simulink model "TormoziRastgard"  (R2014a)
settings: Solver=ode45  StartTime=0.0  StopTime=2  RelTol=1e-3
libraries: powerlib x13, powerlib_meascontrol x1
settings Model: Creator=pc6229  LastModifiedBy=pc6229

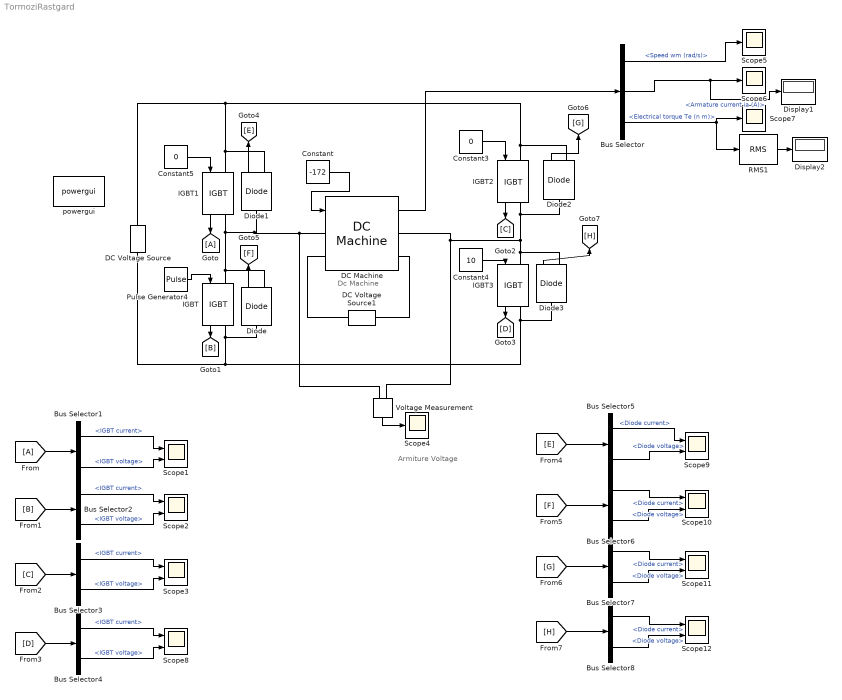
== system TormoziRastgard ==
  note: Armiture Voltage
  note: Dc Machine
  Bus Selector : BusSelector  OutputSignals=Speed wm (rad/s),Armature current ia (A),Electrical torque Te (n m)
  Bus Selector{1..4} (4 alike) : BusSelector  OutputSignals=IGBT current,IGBT voltage
  Bus Selector{5..8} (4 alike) : BusSelector  OutputSignals=Diode current,Diode voltage
  Constant : Constant  Value=-172
  Constant3 : Constant  Value=0
  Constant4 : Constant  Value=10
  Constant5 : Constant  Value=0
  DC Machine : powerlib/Machines/DC Machine  PresetModel=No  MechanicalLoad=Torque TL  FieldType=Wound  ShowDetailedParameters=on  MeasurementBus=off  RLa="[ 0.4  0.04]"  RLf=[ 95 150]  Laf=1.85  MachineConstant=Torque constant (N.m/A)  Ke=1.8  Kt=1.8  J=1  Bm=0  Tf=0  w0=1  Ifinit=1  TsPowergui=0  TsBlock=-1
  DC Voltage Source : powerlib/Electrical Sources/DC Voltage Source  Amplitude=600  Measurements=None
  DC Voltage Source1 : powerlib/Electrical Sources/DC Voltage Source  Amplitude=135  Measurements=None
  Diode{,1..3} (4 alike) : powerlib/Power Electronics/Diode  Ron=0.001  Lon=0  Vf=0.8  IC=0  UseSnubber=off  Rs=500  Cs=250e-9  Measurements=on
  Display1 : Display
  Display2 : Display
  IGBT{,1..3} (4 alike) : powerlib/Power Electronics/IGBT  Ron=0.001  Lon=0  Vf=1  Tf=1e-6  Tt=2e-6  IC=0  Rs=1e5  Cs=inf  Measurements=on
  Pulse Generator4 : DiscretePulseGenerator  PulseType=Time based  Amplitude=10  Period=0.002  PulseWidth=60
  RMS1 : powerlib_meascontrol/Measurements/RMS  TrueRMS=on  Freq=60  RMSInit=120  Ts=0
  Scope{1..3,8..12} (8 alike) : Scope  NumInputPorts=2
      Scope1 settings: YMin=-5~-5  YMax=5~5
      Scope10 settings: YMin=-5~-5  YMax=5~5  SaveName=ScopeData9
      Scope11 settings: YMin=-5~-5  YMax=5~5  SaveName=ScopeData10
      Scope12 settings: YMin=-5~-5  YMax=5~5  SaveName=ScopeData11
      Scope2 settings: YMin=-5~-5  YMax=5~5
      Scope3 settings: YMin=-5~-5  YMax=5~5  SaveName=ScopeData2
      Scope8 settings: YMin=-5~-5  YMax=5~5  SaveName=ScopeData7
      Scope9 settings: YMin=-5~-5  YMax=5~5  SaveName=ScopeData8
  Scope{4..7} (4 alike) : Scope
      Scope4 settings: SaveName=ScopeData3
      Scope5 settings: YMin=100  YMax=107.5  SaveName=ScopeData4
      Scope6 settings: TimeRange=0.01148000060583776  YMin=-90  YMax=10  SaveName=ScopeData5
      Scope7 settings: SaveName=ScopeData6
  Voltage Measurement : powerlib/Measurements/Voltage Measurement  PhasorSimulation=off  OutputType=Complex  PSBequivalent=0
  powergui : powerlib/powergui  Priority=1  SimulationMode=Discrete  SolverType=Tustin  SampleTime=50e-6  frequency=60  SPID=off  DisableSnubberDevices=off  DisableRonSwitches=off  DisableVfSwitches=off  SwTol=0  Interpol=off  DisplayEquations=off  Ts=0  methode=off  frequencyindice=0  Pbase=100e6  ErrMax=1e-4  Iterations=50  UnitsV=kV  UnitsW=MW  FunctionMessages=off  echomessages=off  HookPort=off  EnableUseOfTLC=off  x0status=blocks  RestoreLinks=warning  ResistiveCurrentMeasurement=off  Frange=[0:2:500]  Ylog=off  Xlog=on  ShowGrid=off  save=off  variable=ZData  structure=0  ZoomFFT=off  StartTime=0.0  cycles=1  DisplayStyle=1  fundamental=60  FreqAxis=off  MaxFrequency=1000  frequencyindicesteady=1  RmsSteady=1  display=off
  wires:
  Constant/1 -> DC Machine/1
  DC Machine/1 -> Bus Selector/1
  Bus Selector/1 -> Scope5/1  "<Speed wm (rad/s)>"
  Bus Selector/2 -> Display1/1, Scope6/1  "<Armature current ia (A)>"
  Constant3/1 -> IGBT2/1
  Constant4/1 -> IGBT3/1
  Bus Selector/3 -> RMS1/1, Scope7/1  "<Electrical torque Te (n m)>"
  Pulse Generator4/1 -> IGBT/1
  Constant5/1 -> IGBT1/1
  RMS1/1 -> Display2/1
  Voltage Measurement/1 -> Scope4/1
  IGBT1/1 -> [A]
  IGBT/1 -> [B]
  IGBT2/1 -> [C]
  IGBT3/1 -> [D]
  [A] -> Bus Selector1/1
  [B] -> Bus Selector2/1
  [C] -> Bus Selector3/1
  [D] -> Bus Selector4/1
  Bus Selector1/1 -> Scope1/1  "<IGBT current>"
  Bus Selector1/2 -> Scope1/2  "<IGBT voltage>"
  Bus Selector2/1 -> Scope2/1  "<IGBT current>"
  Bus Selector2/2 -> Scope2/2  "<IGBT voltage>"
  Bus Selector3/2 -> Scope3/2  "<IGBT voltage>"
  Bus Selector3/1 -> Scope3/1  "<IGBT current>"
  Bus Selector4/1 -> Scope8/1  "<IGBT current>"
  Bus Selector4/2 -> Scope8/2  "<IGBT voltage>"
  Diode1/1 -> [E]
  Diode/1 -> [F]
  Diode3/1 -> [H]
  Diode2/1 -> [G]
  [E] -> Bus Selector5/1
  [F] -> Bus Selector6/1
  [G] -> Bus Selector7/1
  [H] -> Bus Selector8/1
  Bus Selector5/1 -> Scope9/1  "<Diode current>"
  Bus Selector5/2 -> Scope9/2  "<Diode voltage>"
  Bus Selector6/1 -> Scope10/1  "<Diode current>"
  Bus Selector6/2 -> Scope10/2  "<Diode voltage>"
  Bus Selector7/1 -> Scope11/1  "<Diode current>"
  Bus Selector7/2 -> Scope11/2  "<Diode voltage>"
  Bus Selector8/1 -> Scope12/1  "<Diode current>"
  Bus Selector8/2 -> Scope12/2  "<Diode voltage>"
  connections:
  DC Voltage Source/RConn1 -- Diode1/RConn1 -- IGBT1/LConn1 -- Diode2/RConn1 -- IGBT2/LConn1
  DC Voltage Source/LConn1 -- Diode/LConn1 -- IGBT/RConn1 -- Diode3/LConn1 -- IGBT3/RConn1
  IGBT/LConn1 -- Voltage Measurement/LConn1 -- DC Machine/LConn1 -- Diode1/LConn1 -- IGBT1/RConn1 -- Diode/RConn1
  DC Machine/RConn1 -- Voltage Measurement/LConn2 -- Diode2/LConn1 -- IGBT2/RConn1 -- Diode3/RConn1 -- IGBT3/LConn1
  DC Voltage Source1/RConn1 -- DC Machine/LConn2
  DC Voltage Source1/LConn1 -- DC Machine/RConn2
